simulink model "DC_MOTOR"  (R2020b)
settings: Solver=VariableStepAuto  StartTime=0.0  StopTime=10.0  RelTol=1e-3
values from neighbouring files (symbols this model uses):
  J = 0.02    [DC_parameters.m]
  Kemf = 0.1    [DC_parameters.m]
  Kf = 0.2    [DC_parameters.m]
  Km = 0.1    [DC_parameters.m]
  L = 0.5    [DC_parameters.m]
  R = 2    [DC_parameters.m]
settings Model: Creator=wangyue  LastModifiedBy=wangyue

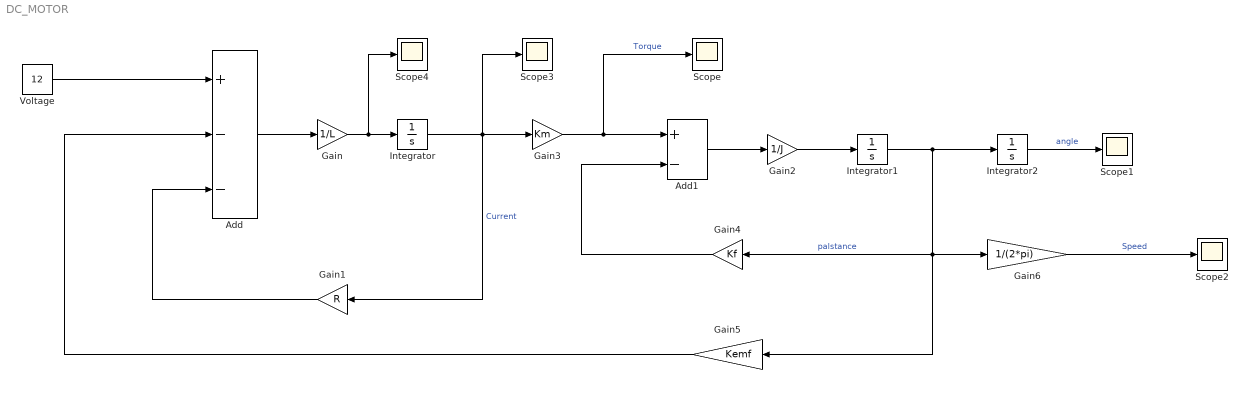
== system DC_MOTOR ==
  Add : Sum  Inputs=+--
  Add1 : Sum  Inputs=+-
  Gain : Gain  Gain=1/L
  Gain1 : Gain  Gain=R
  Gain2 : Gain  Gain=1/J
  Gain3 : Gain  Gain=Km
  Gain4 : Gain  Gain=Kf
  Gain5 : Gain  Gain=Kemf
  Gain6 : Gain  Gain=1/(2*pi)
  Integrator : Integrator
  Integrator1 : Integrator
  Integrator2 : Integrator
  Scope{,1..4} (5 alike) : Scope
  Voltage : Constant  Value=12
  wires:
  Add/1 -> Gain/1
  Voltage/1 -> Add/1
  Gain/1 -> Scope4/1, Integrator/1
  Integrator/1 -> Scope3/1, Gain3/1, Gain1/1  "Current"
  Add1/1 -> Gain2/1
  Gain3/1 -> Scope/1, Add1/1  "Torque"
  Gain2/1 -> Integrator1/1
  Integrator1/1 -> Integrator2/1, Gain6/1, Gain4/1, Gain5/1  "palstance"
  Gain4/1 -> Add1/2
  Gain1/1 -> Add/3
  Gain5/1 -> Add/2
  Integrator2/1 -> Scope1/1  "angle"
  Gain6/1 -> Scope2/1  "Speed"
